simulink library "motor_lib"  (R2020b)
settings: Solver=ode23t  StartTime=0.0  StopTime=10.0  RelTol=1e-3  AbsTol=1e-3  EnableMultiTasking=on
libraries: fl_lib x34, nesl_utility x13, ee_lib x3, simulink x1
settings Model: Creator=scastro  LastModifiedBy=bneiswan
settings SolverCC: AutoScaleAbsTol=off
settings DataIOCC: LimitDataPoints=on  SaveFormat=Array  ReturnWorkspaceOutputs=off
settings OptimizationCC: LifeSpan=inf
settings DebuggingCC: SolverPrmCheckMsg=warning  SFUnexpectedBacktrackingDiag=warning  SFNoUnconditionalDefaultTransitionDiag=warning  SFExecutionAtInitializationDiag=none  ArithmeticOperatorsInVariantConditions=warning
settings HardwareCC: ProdBitPerPointer=32  ProdBitPerSizeT=32  ProdBitPerPtrDiffT=32  ProdLargestAtomicFloat=None  ProdIntDivRoundTo=Undefined  ProdEndianess=Unspecified  ProdWordSize=32  ProdHWDeviceType=32-bit Generic
settings ModelReferenceCC: PropagateSignalLabelsOutOfModel=off
settings SFSimCC: SimUseLocalCustomCode=off
settings RTWCC: RTWUseLocalCustomCode=off
settings CodeAppCC: StateflowObjectComments=on
settings GRTTargetCC: TargetLangStandard=C89/C90 (ANSI)
settings ConfigComp: CovMetricSettings=dw  CovSaveCumulativeToWorkspaceVar=on  CovSaveSingleToWorkspaceVar=on  CovExternalEMLEnable=off  CovSFcnEnable=off

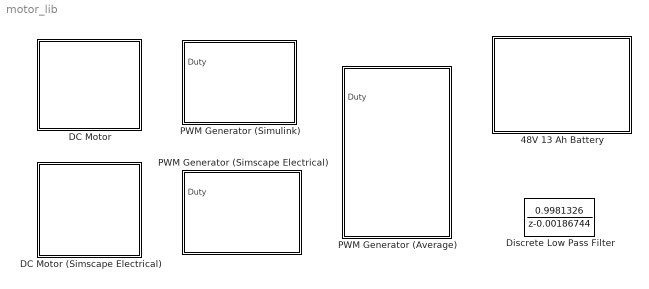
== system motor_lib ==
  48V 13 Ah Battery : Subsystem
      mask Display:
      | image(imread('BatteryIcon.PNG'));
      | color('Orange');
      | port_label('rconn', 1, 'V+');
      | port_label('rconn', 2, 'V-');
  DC Motor : Subsystem
      mask Display:
      | image(imread('MotorIcon.PNG'));
      | color('Orange');
      | port_label('lconn', 1, 'V+');
      | port_label('lconn', 2, 'V-');
      | port_label('rconn', 1, 'R');
      | port_label('rconn', 2, 'C');
  DC Motor (Simscape Electrical) : Subsystem
      mask Display:
      | image(imread('MotorIcon.PNG'));
      | color('Orange');
      | port_label('lconn', 1, 'V+');
      | port_label('lconn', 2, 'V-');
      | port_label('rconn', 1, 'R');
      | port_label('rconn', 2, 'C');
  Discrete Low Pass Filter : DiscreteTransferFcn  Numerator=[0.9981326]  Denominator=[1 -0.00186744]  SampleTime=0.05
  PWM Generator (Average) : Subsystem  mask(PWM Generator){}
      mask help:
      | Average-mode PWM signal generator.
      | The duty cycle input must be a number between 0 and 1.
  PWM Generator (Simscape Electrical) : Subsystem  mask(PWM Generator){freq=50}
      mask prompts: freq "PWM Frequency (Hz)"
      mask help:
      | Average-mode PWM signal generator.
      | The duty cycle input must be a number between 0 and 1.
  PWM Generator (Simulink) : Subsystem  mask(PWM Generator){freq=50, Ts=1e-4}
      mask prompts: freq "PWM Frequency (Hz)"; Ts "Sample Time (s)"
      mask help:
      | Average-mode PWM signal generator.
      | The duty cycle input must be a number between 0 and 1.

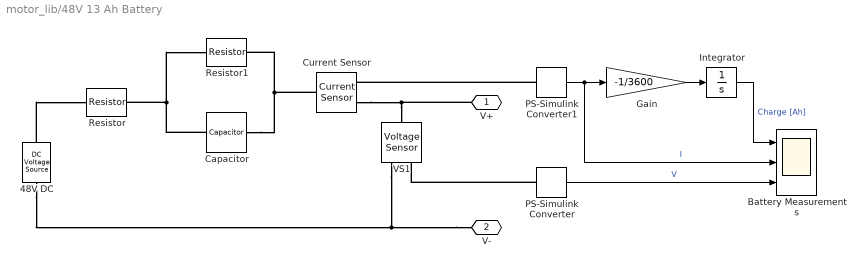
== system motor_lib/48V 13 Ah Battery ==
  48V DC : fl_lib/Electrical/Electrical Sources/DC Voltage Source  v0=48 V
  Battery Measurements : Scope  NumInputPorts=3
  Capacitor : fl_lib/Electrical/Electrical Elements/Capacitor  c=1e-3 F  r=1e-6 Ohm  g=0 1/Ohm  i_specify=off  i_priority=High  i=0 A  i_nominal_specify=off  i_nominal_unit=A  i_nominal_value=1  v_specify=off  v_priority=High  v=0 V  v_nominal_specify=off  v_nominal_unit=V  v_nominal_value=1  vc_specify=on  vc_priority=High  vc=0 V  vc_nominal_specify=off  vc_nominal_unit=V  vc_nominal_value=1
  Current Sensor : fl_lib/Electrical/Electrical Sensors/Current Sensor
  Gain : Gain  Gain=-1/3600
  Integrator : Integrator  InitialCondition=13
      settings: AttributesFormatString=Initial Charge = %<InitialCondition> Ah
  PS-Simulink Converter : nesl_utility/PS-Simulink Converter  PhysicalDomain=network_engine_domain  SubClassName=ps_output  LeftPortType=input  RightPortType=output  PseudoPeriodic=off  Frequencies=[]  Unit=1  AffineConversion=off
  PS-Simulink Converter1 : nesl_utility/PS-Simulink Converter  PhysicalDomain=network_engine_domain  SubClassName=ps_output  LeftPortType=input  RightPortType=output  PseudoPeriodic=off  Frequencies=[]  Unit=1  AffineConversion=off
  Resistor : fl_lib/Electrical/Electrical Elements/Resistor  R=0.07 Ohm  i_specify=off  i_priority=High  i=0 A  i_nominal_specify=off  i_nominal_unit=A  i_nominal_value=1  v_specify=off  v_priority=High  v=0 V  v_nominal_specify=off  v_nominal_unit=V  v_nominal_value=1
  Resistor1 : fl_lib/Electrical/Electrical Elements/Resistor  R=0.05 Ohm  i_specify=off  i_priority=High  i=0 A  i_nominal_specify=off  i_nominal_unit=A  i_nominal_value=1  v_specify=off  v_priority=High  v=0 V  v_nominal_specify=off  v_nominal_unit=V  v_nominal_value=1
  VS1 : fl_lib/Electrical/Electrical Sensors/Voltage Sensor
  V+ : PMIOPort  Side=Right
  V- : PMIOPort  Port=2  Side=Right
  wires:
  PS-Simulink Converter/1 -> Battery Measurements/3  "V"
  PS-Simulink Converter1/1 -> Gain/1, Battery Measurements/2  "I"
  Integrator/1 -> Battery Measurements/1  "Charge [Ah]"
  Gain/1 -> Integrator/1
  connections:
  V-/RConn1 -- 48V DC/RConn1 -- VS1/RConn2
  Resistor1/RConn1 -- Capacitor/RConn1 -- Current Sensor/LConn1
  Resistor/RConn1 -- Capacitor/LConn1 -- Resistor1/LConn1
  VS1/LConn1 -- V+/RConn1 -- Current Sensor/RConn2
  48V DC/LConn1 -- Resistor/LConn1
  PS-Simulink Converter/LConn1 -- VS1/RConn1
  PS-Simulink Converter1/LConn1 -- Current Sensor/RConn1

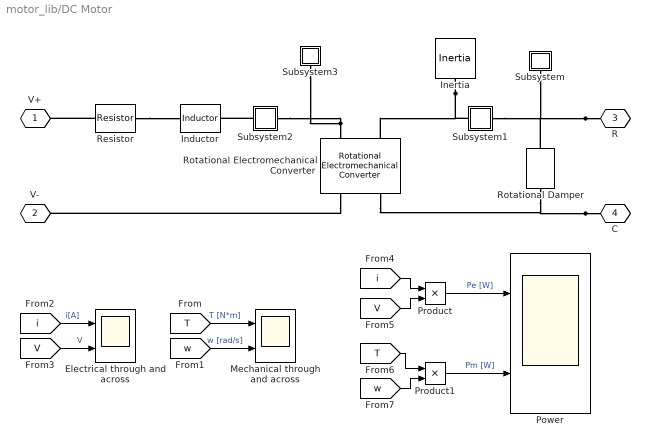
== system motor_lib/DC Motor ==
  Electrical through and across : Scope  NumInputPorts=2
  Inductor : fl_lib/Electrical/Electrical Elements/Inductor  l=1.13e-5 H  r=0 Ohm  g=1e-9 1/Ohm  i_specify=off  i_priority=High  i=0 A  i_nominal_specify=off  i_nominal_unit=A  i_nominal_value=1  v_specify=off  v_priority=High  v=0 V  v_nominal_specify=off  v_nominal_unit=V  v_nominal_value=1  i_L_specify=on  i_L_priority=High  i_L=0 A  i_L_nominal_specify=off  i_L_nominal_unit=A  i_L_nominal_value=1
  Inertia : fl_lib/Mechanical/Rotational Elements/Inertia  inertia=0.01 kg*m^2  num_ports=foundation.enum.numPorts2.one  w_specify=on  w_priority=High  w=0 rad/s  w_nominal_specify=off  w_nominal_unit=rad/s  w_nominal_value=1  t_specify=off  t_priority=High  t=0 N*m  t_nominal_specify=off  t_nominal_unit=N*m  t_nominal_value=1
  Mechanical through and across : Scope  NumInputPorts=2
  Power : Scope  NumInputPorts=2
  Product : Product  RndMeth=Zero
  Product1 : Product  RndMeth=Zero
  Resistor : fl_lib/Electrical/Electrical Elements/Resistor  R=0.750 Ohm  i_specify=off  i_priority=High  i=0 A  i_nominal_specify=off  i_nominal_unit=A  i_nominal_value=1  v_specify=off  v_priority=High  v=0 V  v_nominal_specify=off  v_nominal_unit=V  v_nominal_value=1
  Rotational Electromechanical Converter : fl_lib/Electrical/Electrical Elements/Rotational Electromechanical Converter  K=0.876 V/(rad/s)  i_specify=off  i_priority=High  i=0 A  i_nominal_specify=off  i_nominal_unit=A  i_nominal_value=1  v_specify=off  v_priority=High  v=0 V  v_nominal_specify=off  v_nominal_unit=V  v_nominal_value=1  t_specify=off  t_priority=High  t=0 N*m  t_nominal_specify=off  t_nominal_unit=N*m  t_nominal_value=1  w_specify=off  w_priority=High  w=0 rad/s  w_nominal_specify=off  w_nominal_unit=rad/s  w_nominal_value=1
  Rotational Damper : fl_lib/Mechanical/Rotational Elements/Rotational Damper  D=0.001 N*m/(rad/s)  w_specify=off  w_priority=High  w=0 rad/s  w_nominal_specify=off  w_nominal_unit=rad/s  w_nominal_value=1  t_specify=off  t_priority=High  t=0 N*m  t_nominal_specify=off  t_nominal_unit=N*m  t_nominal_value=1
  Subsystem : Subsystem
      mask Display: disp('w');
  Subsystem1 : Subsystem
      mask Display: disp('T');
  Subsystem2 : Subsystem
      mask Display: disp('i');
  Subsystem3 : Subsystem
      mask Display: disp('V');
  V+ : PMIOPort  Tag=PMCPort  Side=Left
  V- : PMIOPort  Tag=PMCPort  Port=2  Side=Left
  R : PMIOPort  Tag=PMCPort  Port=3  Side=Right
  C : PMIOPort  Tag=PMCPort  Port=4  Side=Right
  wires:
  Product1/1 -> Power/2  "Pm [W]"
  Product/1 -> Power/1  "Pe [W]"
  [w] -> Product1/2
  [T] -> Product1/1
  [V] -> Product/2
  [i] -> Product/1
  [V] -> Electrical through and across/2  "V"
  [i] -> Electrical through and across/1  "i[A]"
  [w] -> Mechanical through and across/2  "w [rad/s]"
  [T] -> Mechanical through and across/1  "T [N*m]"
  connections:
  C/RConn1 -- Rotational Damper/RConn1 -- Rotational Electromechanical Converter/RConn2
  R/RConn1 -- Subsystem/LConn1 -- Rotational Damper/LConn1 -- Subsystem1/RConn1
  Inertia/LConn1 -- Subsystem1/LConn1 -- Rotational Electromechanical Converter/LConn2
  Rotational Electromechanical Converter/LConn1 -- Subsystem3/LConn1 -- Subsystem2/RConn1
  Subsystem2/LConn1 -- Inductor/RConn1
  Resistor/LConn1 -- V+/RConn1
  Rotational Electromechanical Converter/RConn1 -- V-/RConn1
  Resistor/RConn1 -- Inductor/LConn1

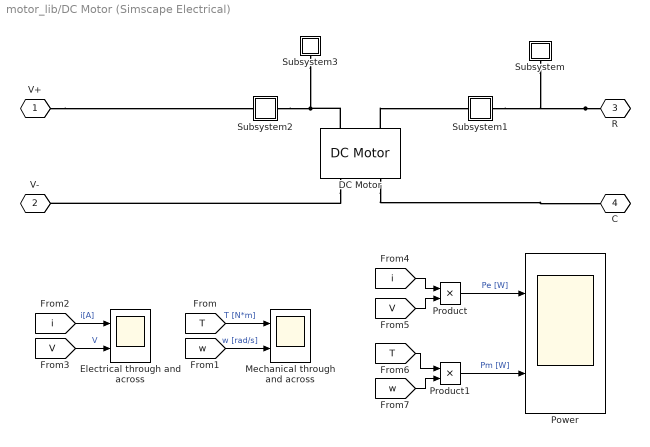
== system motor_lib/DC Motor (Simscape Electrical) ==
  DC Motor : ee_lib/Electromechanical/Brushed Motors/DC Motor  field_option=ee.enum.field_option.pm  Rf=100 Ohm  Lf=1 H  Laf=0.15 H  If0=0 A  parameterization=1  Ra=1 Ohm  La=5e-5 H  emf_or_torque=1  Kv=0.75 V/(rad/s)  Ki=6.876e-4 N*m/A  T_stall=2.4e-4 N*m  w_max=1.91e+4 rpm  w_rated=1.5e+4 rpm  P_rated=0.08 W  V_rated=1.5 V  J=0.01 g*cm^2  lam_param=1  lam=0.001 N*m/(rad/s)  i_noload=0 A  V_i_noload=1.5 V  speed0=0 rpm  enable_fault_armature=ee.enum.faults.faultEnable.no  rev_faulted=1 / 3  G_faulted_armature=1e-5 S  fault_trigger_armature=ee.enum.faults.faultTrigger.temporal  t_fault_armature=1 s  max_permissible_current_armature=inf A  t_fail_on_current_armature=1 s  enable_fault_field=ee.enum.faults.faultEnable.no  G_faulted_field=1e-5 S  fault_trigger_field=ee.enum.faults.faultTrigger.temporal  t_fault_field=1 s  max_permissible_current_field=inf A  t_fail_on_current_field=1 s  fault_action=ee.enum.faults.faultAction.none  alpha=3.93e-3 1/K  Tmeas=25 degC  thermal_mass=100 J/K  initial_temperature=25 degC
  Electrical through and across : Scope  NumInputPorts=2
  Mechanical through and across : Scope  NumInputPorts=2
  Power : Scope  NumInputPorts=2
  Product : Product  RndMeth=Zero
  Product1 : Product  RndMeth=Zero
  Subsystem : Subsystem
      mask Display: disp('w');
  Subsystem1 : Subsystem
      mask Display: disp('T');
  Subsystem2 : Subsystem
      mask Display: disp('i');
  Subsystem3 : Subsystem
      mask Display: disp('V');
  V+ : PMIOPort  Tag=PMCPort  Side=Left
  V- : PMIOPort  Tag=PMCPort  Port=2  Side=Left
  R : PMIOPort  Tag=PMCPort  Port=3  Side=Right
  C : PMIOPort  Tag=PMCPort  Port=4  Side=Right
  wires:
  [T] -> Mechanical through and across/1  "T [N*m]"
  [w] -> Mechanical through and across/2  "w [rad/s]"
  [i] -> Electrical through and across/1  "i[A]"
  [V] -> Electrical through and across/2  "V"
  [i] -> Product/1
  [V] -> Product/2
  [T] -> Product1/1
  [w] -> Product1/2
  Product/1 -> Power/1  "Pe [W]"
  Product1/1 -> Power/2  "Pm [W]"
  connections:
  Subsystem3/LConn1 -- Subsystem2/RConn1 -- DC Motor/LConn1
  R/RConn1 -- Subsystem1/RConn1 -- Subsystem/LConn1
  DC Motor/LConn2 -- Subsystem1/LConn1
  V+/RConn1 -- Subsystem2/LConn1
  DC Motor/RConn2 -- C/RConn1
  DC Motor/RConn1 -- V-/RConn1

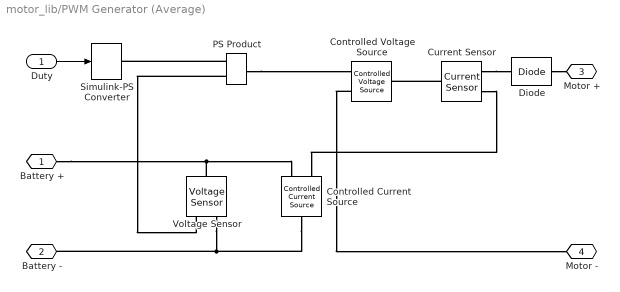
== system motor_lib/PWM Generator (Average) ==
  Duty : Inport
  Controlled Current Source : fl_lib/Electrical/Electrical Sources/Controlled Current Source
  Controlled Voltage Source : fl_lib/Electrical/Electrical Sources/Controlled Voltage Source
  Current Sensor : fl_lib/Electrical/Electrical Sensors/Current Sensor
  Diode : fl_lib/Electrical/Electrical Elements/Diode  Vf=1e-3 V  Ron=1e-3 Ohm  Goff=1e-8 1/Ohm  i_specify=off  i_priority=None  i=0 A  i_nominal_specify=off  i_nominal_unit=A  i_nominal_value=1  v_specify=off  v_priority=None  v=0 V  v_nominal_specify=off  v_nominal_unit=V  v_nominal_value=1
  PS Product : fl_lib/Physical Signals/Functions/PS Product
  Simulink-PS Converter : nesl_utility/Simulink-PS Converter  PhysicalDomain=network_engine_domain  SubClassName=ps_input  LeftPortType=input  RightPortType=output  PseudoPeriodic=off  Frequencies=[]  NoiseDistribution=none  NoiseParameters=[]  Unit=1  AffineConversion=off  FilteringAndDerivatives=zero  SimscapeFilterOrder=1  InputFilterTimeConstant=0.001  UdotUserProvided=1
  Voltage Sensor : fl_lib/Electrical/Electrical Sensors/Voltage Sensor
  Battery + : PMIOPort  Side=Left
  Battery - : PMIOPort  Port=2  Side=Left
  Motor + : PMIOPort  Port=3  Side=Right
  Motor - : PMIOPort  Port=4  Side=Right
  wires:
  Duty/1 -> Simulink-PS Converter/1
  connections:
  Current Sensor/LConn1 -- Controlled Voltage Source/LConn1
  Controlled Voltage Source/RConn2 -- Motor -/RConn1
  Current Sensor/RConn1 -- Controlled Current Source/RConn1
  PS Product/LConn2 -- Voltage Sensor/RConn1
  Voltage Sensor/LConn1 -- Controlled Current Source/RConn2 -- Battery +/RConn1
  PS Product/RConn1 -- Controlled Voltage Source/RConn1
  Current Sensor/RConn2 -- Diode/LConn1
  PS Product/LConn1 -- Simulink-PS Converter/RConn1
  Voltage Sensor/RConn2 -- Controlled Current Source/LConn1 -- Battery -/RConn1
  Diode/RConn1 -- Motor +/RConn1

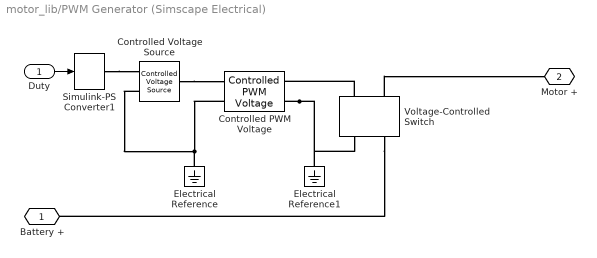
== system motor_lib/PWM Generator (Simscape Electrical) ==
  Duty : Inport
  Controlled PWM Voltage : ee_lib/Integrated Circuits/Controlled PWM Voltage  F=freq Hz  TD=0 s  pulse_width_offset=0 s  pulse_min=0 s  Vmin=0 V  Vmax=1 V  Vm=1 V  pwm_or_av=1  event_type=1  sample_time=1e-6 s  u_min=0  u_max=1
  Controlled Voltage Source : fl_lib/Electrical/Electrical Sources/Controlled Voltage Source
  Electrical Reference : fl_lib/Electrical/Electrical Elements/Electrical Reference
  Electrical Reference1 : fl_lib/Electrical/Electrical Elements/Electrical Reference
  Simulink-PS Converter1 : nesl_utility/Simulink-PS Converter  PhysicalDomain=network_engine_domain  SubClassName=ps_input  LeftPortType=input  RightPortType=output  PseudoPeriodic=off  Frequencies=[]  NoiseDistribution=none  NoiseParameters=[]  Unit=V  AffineConversion=off  FilteringAndDerivatives=zero  SimscapeFilterOrder=1  InputFilterTimeConstant=0.001  UdotUserProvided=1
  Voltage-Controlled Switch : ee_lib/Additional Components/SPICE Passives/Voltage-Controlled Switch  SWITCH_model=ee.enum.switches.switchModelVoltage.transition  VON=1 V  VOFF=0 V  VT=1e-3 V  VH=0 V  RON=1e-3 Ohm  ROFF_res=1e6 Ohm  Roff_gmin=ee.enum.switches.offResistance.no  ROFF=1e8 Ohm  TD=0 s
      settings: SourceProductBaseCode=PS  InternalSimscapePortConfiguration="{\"Bottom\":[],\"Left\":[{\"id\":\"p1\",\"label\":\"1+\",\"type\":\"foundation.electrical.electrical\"},{\"id\":\"p2\",\"label\":\"2+\",\"type\":\"foundation.electrical.electrical\"}],\"Right\":[{\"id\":\"n1\",\"label\":\"1-\",\"type\":\"foundation.electrical.electrical\"},{\"id\":\"n2\",\"label\":\"2-\",\"type\":\"foundation.electrical.electrical\"}],\"Top\":[]}"
  Battery + : PMIOPort  Side=Left
  Motor + : PMIOPort  Port=2  Side=Right
  wires:
  Duty/1 -> Simulink-PS Converter1/1
  connections:
  Electrical Reference/LConn1 -- Controlled Voltage Source/RConn2 -- Controlled PWM Voltage/LConn2
  Controlled PWM Voltage/RConn2 -- Electrical Reference1/LConn1 -- Voltage-Controlled Switch/RConn1
  Voltage-Controlled Switch/LConn1 -- Controlled PWM Voltage/RConn1
  Voltage-Controlled Switch/RConn2 -- Battery +/RConn1
  Voltage-Controlled Switch/LConn2 -- Motor +/RConn1
  Simulink-PS Converter1/RConn1 -- Controlled Voltage Source/RConn1
  Controlled Voltage Source/LConn1 -- Controlled PWM Voltage/LConn1

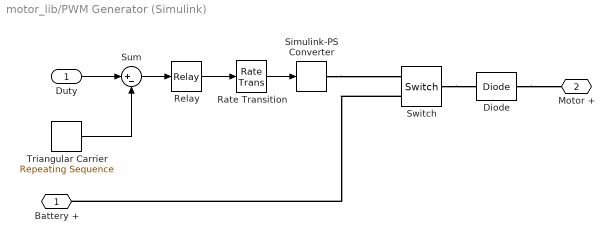
== system motor_lib/PWM Generator (Simulink) ==
  Duty : Inport
  Diode : fl_lib/Electrical/Electrical Elements/Diode  Vf=1e-3 V  Ron=1e-3 Ohm  Goff=1e-8 1/Ohm  i_specify=off  i_priority=None  i=0 A  i_nominal_specify=off  i_nominal_unit=A  i_nominal_value=1  v_specify=off  v_priority=None  v=0 V  v_nominal_specify=off  v_nominal_unit=V  v_nominal_value=1
  Rate Transition : RateTransition  OutPortSampleTime=Ts
  Relay : Relay  OnSwitchValue=1e-6  OffSwitchValue=1e-6
  Simulink-PS Converter : nesl_utility/Simulink-PS Converter  PhysicalDomain=network_engine_domain  SubClassName=ps_input  LeftPortType=input  RightPortType=output  PseudoPeriodic=off  Frequencies=[]  NoiseDistribution=none  NoiseParameters=[]  Unit=1  AffineConversion=off  FilteringAndDerivatives=zero  SimscapeFilterOrder=1  InputFilterTimeConstant=0.001  UdotUserProvided=1
  Sum : Sum  Inputs=|+-
  Switch : fl_lib/Electrical/Electrical Elements/Switch  R_closed=0.01 Ohm  G_open=1e-8 1/Ohm  Threshold=0  i_specify=off  i_priority=None  i=0 A  i_nominal_specify=off  i_nominal_unit=A  i_nominal_value=1  v_specify=off  v_priority=None  v=0 V  v_nominal_specify=off  v_nominal_unit=V  v_nominal_value=1
  Triangular Carrier : simulink/Sources/Repeating Sequence  rep_seq_t=[0 1/freq]  rep_seq_y=[0 1]
  Battery + : PMIOPort  Side=Left
  Motor + : PMIOPort  Port=2  Side=Right
  wires:
  Rate Transition/1 -> Simulink-PS Converter/1
  Relay/1 -> Rate Transition/1
  Triangular Carrier/1 -> Sum/2
  Sum/1 -> Relay/1
  Duty/1 -> Sum/1
  connections:
  Diode/RConn1 -- Motor +/RConn1
  Switch/RConn2 -- Battery +/RConn1
  Simulink-PS Converter/RConn1 -- Switch/RConn1
  Switch/LConn1 -- Diode/LConn1

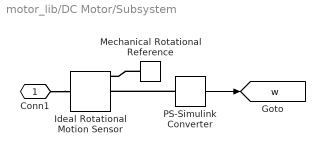
== system motor_lib/DC Motor/Subsystem ==
  Ideal Rotational Motion Sensor : fl_lib/Mechanical/Mechanical Sensors/Ideal Rotational Motion Sensor  wrap_angle=simscape.enum.onoff.off  offset=0 rad
  Mechanical Rotational Reference : fl_lib/Mechanical/Rotational Elements/Mechanical Rotational Reference
  PS-Simulink Converter : nesl_utility/PS-Simulink Converter  PhysicalDomain=network_engine_domain  SubClassName=ps_output  LeftPortType=input  RightPortType=output  PseudoPeriodic=off  Frequencies=[]  Unit=rad/s  AffineConversion=off
  Conn1 : PMIOPort  Side=Left
  tag scope: w=global
  wires:
  PS-Simulink Converter/1 -> [w]
  connections:
  Mechanical Rotational Reference/LConn1 -- Ideal Rotational Motion Sensor/RConn1
  Conn1/RConn1 -- Ideal Rotational Motion Sensor/LConn1
  PS-Simulink Converter/LConn1 -- Ideal Rotational Motion Sensor/RConn2

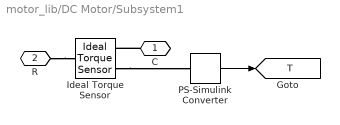
== system motor_lib/DC Motor/Subsystem1 ==
  Ideal Torque Sensor : fl_lib/Mechanical/Mechanical Sensors/Ideal Torque Sensor
  PS-Simulink Converter : nesl_utility/PS-Simulink Converter  PhysicalDomain=network_engine_domain  SubClassName=ps_output  LeftPortType=input  RightPortType=output  PseudoPeriodic=off  Frequencies=[]  Unit=N*m  AffineConversion=off
  C : PMIOPort  Side=Right
  R : PMIOPort  Port=2  Side=Left
  tag scope: T=global
  wires:
  PS-Simulink Converter/1 -> [T]
  connections:
  Ideal Torque Sensor/RConn2 -- PS-Simulink Converter/LConn1
  C/RConn1 -- Ideal Torque Sensor/RConn1
  R/RConn1 -- Ideal Torque Sensor/LConn1

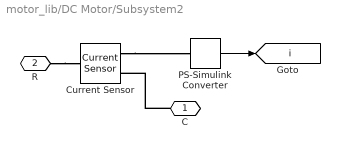
== system motor_lib/DC Motor/Subsystem2 ==
  Current Sensor : fl_lib/Electrical/Electrical Sensors/Current Sensor
  PS-Simulink Converter : nesl_utility/PS-Simulink Converter  PhysicalDomain=network_engine_domain  SubClassName=ps_output  LeftPortType=input  RightPortType=output  PseudoPeriodic=off  Frequencies=[]  Unit=A  AffineConversion=off
  C : PMIOPort  Side=Right
  R : PMIOPort  Port=2  Side=Left
  tag scope: i=global
  wires:
  PS-Simulink Converter/1 -> [i]
  connections:
  Current Sensor/RConn1 -- PS-Simulink Converter/LConn1
  C/RConn1 -- Current Sensor/RConn2
  R/RConn1 -- Current Sensor/LConn1

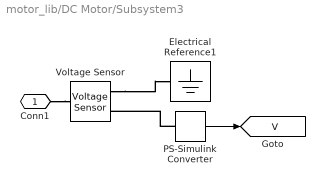
== system motor_lib/DC Motor/Subsystem3 ==
  Electrical Reference1 : fl_lib/Electrical/Electrical Elements/Electrical Reference
  PS-Simulink Converter : nesl_utility/PS-Simulink Converter  PhysicalDomain=network_engine_domain  SubClassName=ps_output  LeftPortType=input  RightPortType=output  PseudoPeriodic=off  Frequencies=[]  Unit=V  AffineConversion=off
  Voltage Sensor : fl_lib/Electrical/Electrical Sensors/Voltage Sensor
  Conn1 : PMIOPort  Side=Left
  tag scope: V=global
  wires:
  PS-Simulink Converter/1 -> [V]
  connections:
  Voltage Sensor/RConn2 -- Electrical Reference1/LConn1
  Conn1/RConn1 -- Voltage Sensor/LConn1
  PS-Simulink Converter/LConn1 -- Voltage Sensor/RConn1

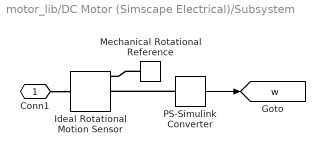
== system motor_lib/DC Motor (Simscape Electrical)/Subsystem ==
  Ideal Rotational Motion Sensor : fl_lib/Mechanical/Mechanical Sensors/Ideal Rotational Motion Sensor  wrap_angle=simscape.enum.onoff.off  offset=0 rad
  Mechanical Rotational Reference : fl_lib/Mechanical/Rotational Elements/Mechanical Rotational Reference
  PS-Simulink Converter : nesl_utility/PS-Simulink Converter  PhysicalDomain=network_engine_domain  SubClassName=ps_output  LeftPortType=input  RightPortType=output  PseudoPeriodic=off  Frequencies=[]  Unit=rad/s  AffineConversion=off
  Conn1 : PMIOPort  Side=Left
  tag scope: w=global
  wires:
  PS-Simulink Converter/1 -> [w]
  connections:
  PS-Simulink Converter/LConn1 -- Ideal Rotational Motion Sensor/RConn2
  Conn1/RConn1 -- Ideal Rotational Motion Sensor/LConn1
  Mechanical Rotational Reference/LConn1 -- Ideal Rotational Motion Sensor/RConn1

== system motor_lib/DC Motor (Simscape Electrical)/Subsystem1 ==
  Ideal Torque Sensor : fl_lib/Mechanical/Mechanical Sensors/Ideal Torque Sensor
  PS-Simulink Converter : nesl_utility/PS-Simulink Converter  PhysicalDomain=network_engine_domain  SubClassName=ps_output  LeftPortType=input  RightPortType=output  PseudoPeriodic=off  Frequencies=[]  Unit=N*m  AffineConversion=off
  C : PMIOPort  Side=Right
  R : PMIOPort  Port=2  Side=Left
  tag scope: T=global
  wires:
  PS-Simulink Converter/1 -> [T]
  connections:
  R/RConn1 -- Ideal Torque Sensor/LConn1
  C/RConn1 -- Ideal Torque Sensor/RConn1
  Ideal Torque Sensor/RConn2 -- PS-Simulink Converter/LConn1

== system motor_lib/DC Motor (Simscape Electrical)/Subsystem2 ==
  Current Sensor : fl_lib/Electrical/Electrical Sensors/Current Sensor
  PS-Simulink Converter : nesl_utility/PS-Simulink Converter  PhysicalDomain=network_engine_domain  SubClassName=ps_output  LeftPortType=input  RightPortType=output  PseudoPeriodic=off  Frequencies=[]  Unit=A  AffineConversion=off
  C : PMIOPort  Side=Right
  R : PMIOPort  Port=2  Side=Left
  tag scope: i=global
  wires:
  PS-Simulink Converter/1 -> [i]
  connections:
  R/RConn1 -- Current Sensor/LConn1
  C/RConn1 -- Current Sensor/RConn2
  Current Sensor/RConn1 -- PS-Simulink Converter/LConn1

== system motor_lib/DC Motor (Simscape Electrical)/Subsystem3 ==
  Electrical Reference1 : fl_lib/Electrical/Electrical Elements/Electrical Reference
  PS-Simulink Converter : nesl_utility/PS-Simulink Converter  PhysicalDomain=network_engine_domain  SubClassName=ps_output  LeftPortType=input  RightPortType=output  PseudoPeriodic=off  Frequencies=[]  Unit=V  AffineConversion=off
  Voltage Sensor : fl_lib/Electrical/Electrical Sensors/Voltage Sensor
  Conn1 : PMIOPort  Side=Left
  tag scope: V=global
  wires:
  PS-Simulink Converter/1 -> [V]
  connections:
  PS-Simulink Converter/LConn1 -- Voltage Sensor/RConn1
  Conn1/RConn1 -- Voltage Sensor/LConn1
  Voltage Sensor/RConn2 -- Electrical Reference1/LConn1
